simulink model "ball"  (R2016a)
settings: Solver=FixedStepDiscrete  StartTime=0.0  StopTime=inf  FixedStep=0.1  RelTol=1e-3
settings Model: Creator=DELL  LastModifiedBy=DELL
settings SolverCC: AutoInsertRateTranBlk=on
settings DataIOCC: LimitDataPoints=on
settings DebuggingCC: AllowSymbolicDim=off
settings ConfigComp: CovModelRefEnable=Off  CovSFcnEnable=off

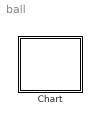
== system ball ==
  Chart : Stateflow chart  TreatAsAtomicUnit=on

== stateflow chart ball/Chart ==
  state a7
    entry: a=uint8(7*rand(1));
  state a6
    entry: a=uint8(7*rand(1));
  state a0
    entry: x=uint8(7*rand(1));
  state a5
    entry: s=uint8(7*rand(1));
  state a1
    entry: y=uint8(7*rand(1));
  state a4
    entry: s=uint8(7*rand(1));
  state a2
    entry: z=uint8(7*rand(1));
  state a3
    entry: a=uint8(7*rand(1));
  a6 -> a6 [order 1] : [a==9]
  a7 -> a7 [order 1] : [a==0]
  (default) -> a7
  a0 -> a6 [order 2] : [x==1]
  a0 -> a7 [order 1] : [x==0]
  a6 -> a0 [order 3] : [s==2]
  a7 -> a0 [order 2] : [a==1]
  a6 -> a1 [order 4] : [s==3]
  a7 -> a1 [order 3] : [a==2]
  a1 -> a7 [order 7] : [y==6]
  a1 -> a6 [order 6] : [y==5]
  a7 -> a6 [order 8] : [a==7]
  a7 -> a4 [order 6] : [a==5]
  a2 -> a7 [order 6] : [z==6]
  a6 -> a7 [order 2] : [s==1]
  a2 -> a6 [order 5] : [z==5]
  a7 -> a5 [order 7] : [a==6]
  a7 -> a3 [order 5] : [a==4]
  a6 -> a2 [order 5] : [s==4]
  a7 -> a2 [order 4] : [a==3]
  a4 -> a7 [order 4] : [s==3]
  a3 -> a7 [order 5] : [a==4]
  a5 -> a7 [order 3] : [s==2]
  a6 -> a4 [order 7] : [s==6]
  a6 -> a3 [order 6] : [s==5]
  a3 -> a6 [order 4] : [a==3]
  a6 -> a5 [order 8] : [s==7]
  a4 -> a6 [order 3] : [s==2]
  a5 -> a6 [order 2] : [s==1]
  a1 -> a0 [order 8] : [y==7]
  a0 -> a0 [order 8] : [x==7]
  a5 -> a5 [order 1] : [s==0]
  a0 -> a5 [order 3] : [x==2]
  a3 -> a0 [order 6] : [a==5]
  a4 -> a5 [order 2] : [s==1]
  a0 -> a4 [order 4] : [x==3]
  a5 -> a0 [order 4] : [s==3]
  a4 -> a0 [order 5] : [s==4]
  a5 -> a3 [order 7] : [s==6]
  a0 -> a3 [order 5] : [x==4]
  a1 -> a5 [order 5] : [y==4]
  a0 -> a2 [order 6] : [x==5]
  a5 -> a1 [order 5] : [s==4]
  a2 -> a0 [order 8] : [z==7]
  a3 -> a5 [order 3] : [a==2]
  a5 -> a4 [order 8] : [s==7]
  a0 -> a1 [order 7] : [x==6]
  a5 -> a2 [order 6] : [s==5]
  a2 -> a5 [order 4] : [z==3]
  a3 -> a1 [order 7] : [a==6]
  a4 -> a1 [order 6] : [s==5]
  a1 -> a1 [order 1] : [y==0]
  a4 -> a3 [order 8] : [s==7]
  a1 -> a3 [order 3] : [y==2]
  a4 -> a2 [order 7] : [s==6]
  a1 -> a2 [order 2] : [y==1]
  a4 -> a4 [order 1] : [s==0]
  a1 -> a4 [order 4] : [y==3]
  a2 -> a4 [order 3] : [z==1]
  a3 -> a4 [order 2] : [a==0]
  a2 -> a3 [order 2] : [z==2]
  a2 -> a1 [order 7] : [z==4]
  a3 -> a2 [order 8] : [a==7]
  a2 -> a2 [order 1] : [z==0]
  a3 -> a3 [order 1] : [a==1]
  data: x local; z local; a local; s local; y local
